simulink library "Lib_PFSys_Capacitor_TMATS"  (R2018a)
settings: Solver=ode45  StartTime=0.0  StopTime=10.0  RelTol=1e-3  EnableMultiTasking=on
libraries: Lib_PF_BusLoadDC_TMATS x1, Lib_PF_LineDC_TMATS x1
Description:
  | Thomas Modules
settings Model: Creator=jwchapm2  LastModifiedBy=mebell
settings DataIOCC: LimitDataPoints=on  SaveFormat=Array
settings OptimizationCC: ExpressionDepthLimit=2147483647  LifeSpan=inf
settings DebuggingCC: UnderspecifiedInitializationDetection=Classic  MergeDetectMultiDrivingBlocksExec=none  SolverPrmCheckMsg=warning  StateNameClashWarn=warning  SFUnexpectedBacktrackingDiag=warning  SFNoUnconditionalDefaultTransitionDiag=warning  SFExecutionAtInitializationDiag=none
settings HardwareCC: ProdBitPerPointer=32  ProdBitPerSizeT=32  ProdBitPerPtrDiffT=32  ProdLargestAtomicFloat=None  ProdIntDivRoundTo=Undefined  ProdEndianess=Unspecified  ProdWordSize=32  ProdHWDeviceType=32-bit Generic
settings ModelReferenceCC: PropagateSignalLabelsOutOfModel=off
settings CodeAppCC: StateflowObjectComments=on
settings GRTTargetCC: TargetLangStandard=C89/C90 (ANSI)  GeneratePreprocessorConditionals=Disable all
settings ConfigComp: CovMetricSettings=dw  CovHtmlReporting=on  CovSaveCumulativeToWorkspaceVar=on  CovSaveSingleToWorkspaceVar=on  CovExternalEMLEnable=off

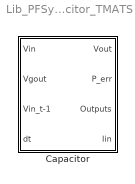
== system Lib_PFSys_Capacitor_TMATS ==
  Capacitor : Subsystem  mask(Capacitor){C_M=100e-6, ESR_M=0.001, I_Leak_M=1e-5}
      mask prompts: C_M "C_M - Capacitance, Farads"; ESR_M "ESR_M - Equivalent series resistance, Ohms"; I_Leak_M "I_Leak_M - Leakage current, Amps"
      mask help: This block represents a capacitor, with a specified capacitance (C_M, in Farads), equivalent series resistance (ESR_M, in Ohms), and constant leakage curent (I_Leak_M, in Amps).

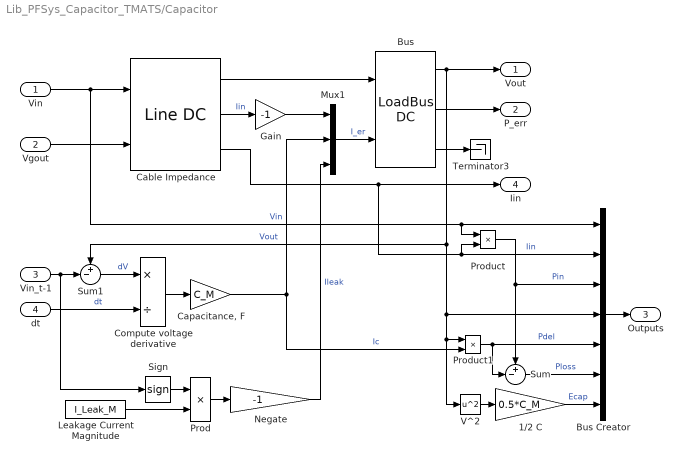
== system Lib_PFSys_Capacitor_TMATS/Capacitor ==
  Vin : Inport
  Vgout : Inport  Port=2
  Vin_t-1 : Inport  Port=3
  dt : Inport  Port=4
  1/2 C : Gain  Gain=0.5*C_M
  Bus : Lib_PF_BusLoadDC_TMATS/LoadBus DC  PeInEN_M=off  P_M=0  BlkNm_M=double(gcb)
  Bus Creator : BusCreator  Inputs=7
  Cable Impedance : Lib_PF_LineDC_TMATS/Line DC  R_M=ESR_M
  "Capacitance, F" : Gain  Gain=C_M
  Compute voltage derivative : Product  Inputs=*/
  Gain : Gain  Gain=-1
  Leakage Current Magnitude : Constant  Value=I_Leak_M
  Mux1 : Mux  Inputs=3
  Negate : Gain  Gain=-1
  Prod : Product  Inputs=**
  Product : Product
  Product1 : Product
  Sign : Signum
  Sum : Sum  Inputs=+-|
  Sum1 : Sum  Inputs=+-|
  Terminator3 : Terminator
  V^2 : Math  Operator=square  SaturateOnIntegerOverflow=on
  Vout : Outport
  P_err : Outport  Port=2
  Outputs : Outport  Port=3
  Iin : Outport  Port=4
  wires:
  Sum/1 -> Bus Creator/6  "Ploss"
  Bus/1 -> Vout/1, Sum1/1, Bus Creator/4, V^2/1, Product1/1  "Vout"
  Product1/1 -> Sum/2, Bus Creator/5  "Pdel"
  Cable Impedance/3 -> Bus Creator/2, Product/2, Iin/1  "Iin"
  Bus Creator/1 -> Outputs/1
  Vin/1 -> Cable Impedance/1, Bus Creator/1, Product/1  "Vin"
  Product/1 -> Bus Creator/3, Sum/1  "Pin"
  Bus/3 -> Terminator3/1
  Bus/2 -> P_err/1
  Mux1/1 -> Bus/2  "I_er"
  Leakage Current Magnitude/1 -> Prod/2
  Sign/1 -> Prod/1
  Prod/1 -> Negate/1
  1/2 C/1 -> Bus Creator/7  "Ecap"
  V^2/1 -> 1/2 C/1
  Negate/1 -> Mux1/3  "Ileak"
  Vin_t-1/1 -> Sign/1, Sum1/2
  Compute voltage derivative/1 -> "Capacitance, F"/1
  dt/1 -> Compute voltage derivative/2  "dt"
  "Capacitance, F"/1 -> Product1/2, Mux1/2  "Ic"
  Sum1/1 -> Compute voltage derivative/1  "dV"
  Cable Impedance/2 -> Gain/1  "Iin"
  Vgout/1 -> Cable Impedance/2
  Cable Impedance/1 -> Bus/1
  Gain/1 -> Mux1/1
